simulink model "HouseHolderTransformTest"  (R2023b)
settings: Solver=VariableStepAuto  StartTime=0.0  StopTime=1  FixedStep=0.0038461538461538464  RelTol=1e-3
values from neighbouring files (symbols this model uses):
  A = [0.588528123101 -3.46944695195e-18 -8.67361737988e-19 0 0 6.93889390391e-18 6.93889390391e-18 6.93889390391e-18 1.38777878078e-17 0 0 6.93889390391e-18 ... (1040 elements, 260x4)]    [InitData.mat]
undefined symbols (not defined in the file or in its folder): FrameLength, NumOfAntennas
libraries: hdlsllib x5, dspstat3 x5
(part 2 of 2)

== system HouseHolderTransformTest/Subsystem/Subsystem3/vecnorm(A(k:end, k:end), 2, 1)/For Iterator Subsystem ==
  input : Inport
  N : Inport  Port=2
  2nd Norm : Subsystem
  Assignment : Assignment  IndexOptions=Index vector (port)  Indices=1  OutputSizes=1
  Constant : Constant  Value=zeros(1 , NumOfAntennas)
  For Iterator : ForIterator  IterationSource=external
  Selector : Selector  NumberOfDimensions=2  InputPortWidth=3  IndexOptions=Select all,Index vector (port)  Indices=[1 3],1  OutputSizes=1,1
  output : Outport
  wires:
  Assignment/1 -> output/1
  2nd Norm/1(output) -> Assignment/2
  Constant/1 -> Assignment/1
  N/1 -> For Iterator/1
  Selector/1 -> 2nd Norm/1(input)
  For Iterator/1 -> Selector/2, Assignment/3
  input/1 -> Selector/1

== system HouseHolderTransformTest/Subsystem/Subsystem4/BLOCK B/2nd Norm ==
  input : Inport
  Add : Sum
  Complex to Real-Imag : ComplexToRealImag
  Sqrt : Sqrt
  Square : Math  Operator=square  SignedPower=on  RndMeth=Zero
  Square1 : Math  Operator=square  SignedPower=on  RndMeth=Zero
  Sum of Elements : Sum  Inputs=+
  output : Outport
  wires:
  input/1 -> Complex to Real-Imag/1
  Complex to Real-Imag/2 -> Square1/1
  Sqrt/1 -> output/1
  Complex to Real-Imag/1 -> Square/1
  Square/1 -> Add/1
  Add/1 -> Sum of Elements/1
  Sum of Elements/1 -> Sqrt/1
  Square1/1 -> Add/2

== system HouseHolderTransformTest/Subsystem/Subsystem4/BLOCK B/If Action Subsystem ==
  norm : Inport
  x : Inport  Port=2
  Assignment : Assignment  IndexOptions=Index vector (dialog)  Indices=1  OutputSizes=1
  Divide : Subsystem  Tag=DecoupledSystem
  Divide1 : Subsystem  Tag=DecoupledSystem
  Selector : Selector  NumberOfDimensions=2  InputPortWidth=FrameLength  IndexOptions=Starting index (dialog),Index vector (dialog)  Indices=1,1  OutputSizes=1,1
  Sqrt : Sqrt
  Subsystem Reference : Subsystem  ReferencedSubsystem=CompAbs
  getU(1) : Subsystem
  u : Outport
  wires:
  getU(1)/1(u(1)) -> Subsystem Reference/1, Assignment/2  "u1"
  Assignment/1 -> Divide1/1(In1)
  Subsystem Reference/1 -> Sqrt/1
  Divide1/1(Out1) -> u/1
  Divide/1(Out1) -> Assignment/1, Selector/1
  norm/1 -> Divide/2(In2)
  x/1 -> Divide/1(In1)
  Selector/1 -> getU(1)/1(input)  "u1"
  Sqrt/1 -> Divide1/2(In2)

== system HouseHolderTransformTest/Subsystem/Subsystem4/BLOCK B/If Action Subsystem1 ==
  x : Inport
  Assignment : Assignment  IndexOptions=Index vector (dialog)  Indices=1  OutputSizes=1
  Constant : Constant  Value=sqrt(2)
  u : Outport
  wires:
  Assignment/1 -> u/1
  Constant/1 -> Assignment/2
  x/1 -> Assignment/1

== system HouseHolderTransformTest/Subsystem/Subsystem4/vecnorm(A(k:end, k:end), 2, 1)/For Iterator Subsystem ==
  input : Inport
  N : Inport  Port=2
  2nd Norm : Subsystem
  Assignment : Assignment  IndexOptions=Index vector (port)  Indices=1  OutputSizes=1
  Constant : Constant  Value=zeros(1 , NumOfAntennas)
  For Iterator : ForIterator  IterationSource=external
  Selector : Selector  NumberOfDimensions=2  InputPortWidth=3  IndexOptions=Select all,Index vector (port)  Indices=[1 3],1  OutputSizes=1,1
  output : Outport
  wires:
  input/1 -> Selector/1
  For Iterator/1 -> Assignment/3, Selector/2
  Selector/1 -> 2nd Norm/1(input)
  N/1 -> For Iterator/1
  Constant/1 -> Assignment/1
  2nd Norm/1(output) -> Assignment/2
  Assignment/1 -> output/1

== system HouseHolderTransformTest/For Iterator Subsystem1/Subsystem3/BLOCK B/If Action Subsystem/Divide ==
  In1 : Inport  LockScale=on
  In2 : Inport  Port=2  LockScale=on
  DTC_input_1 : DataTypeConversion  OutDataTypeStr=fixdt('double')  RndMeth=Nearest  SaturateOnIntegerOverflow=off  LockScale=on
  DTC_input_2 : DataTypeConversion  OutDataTypeStr=fixdt('double')  RndMeth=Nearest  SaturateOnIntegerOverflow=off  LockScale=on
  DTC_output_1 : DataTypeConversion  OutDataTypeStr=fixdt('double')  SaturateOnIntegerOverflow=off  RndMeth=Floor
  ReplicaOfSource : Product  Inputs=*/  RndMeth=Zero  SaturateOnIntegerOverflow=on
  Out1 : Outport  LockScale=on
  wires:
  ReplicaOfSource/1 -> DTC_output_1/1
  In1/1 -> DTC_input_1/1
  DTC_output_1/1 -> Out1/1
  In2/1 -> DTC_input_2/1
  DTC_input_2/1 -> ReplicaOfSource/2
  DTC_input_1/1 -> ReplicaOfSource/1

== system HouseHolderTransformTest/For Iterator Subsystem1/Subsystem3/BLOCK B/If Action Subsystem/Divide1 ==
  In1 : Inport  LockScale=on
  In2 : Inport  Port=2  LockScale=on
  DTC_input_1 : DataTypeConversion  OutDataTypeStr=fixdt('double')  RndMeth=Nearest  SaturateOnIntegerOverflow=off  LockScale=on
  DTC_input_2 : DataTypeConversion  OutDataTypeStr=fixdt('double')  RndMeth=Nearest  SaturateOnIntegerOverflow=off  LockScale=on
  DTC_output_1 : DataTypeConversion  OutDataTypeStr=fixdt('double')  SaturateOnIntegerOverflow=off  RndMeth=Floor
  ReplicaOfSource : Product  Inputs=*/  RndMeth=Zero  SaturateOnIntegerOverflow=on
  Out1 : Outport  LockScale=on
  wires:
  DTC_output_1/1 -> Out1/1
  In2/1 -> DTC_input_2/1
  In1/1 -> DTC_input_1/1
  DTC_input_1/1 -> ReplicaOfSource/1
  ReplicaOfSource/1 -> DTC_output_1/1
  DTC_input_2/1 -> ReplicaOfSource/2

== system HouseHolderTransformTest/For Iterator Subsystem1/Subsystem3/BLOCK B/If Action Subsystem/getU(1) ==
  input : Inport
  Add1 : Sum
  signNonComplex : Subsystem
  u(1) : Outport
  wires:
  signNonComplex/1(Out1) -> Add1/1
  input/1 -> Add1/2, signNonComplex/1(input)
  Add1/1 -> u(1)/1  "u(1)"

== system HouseHolderTransformTest/For Iterator Subsystem1/Subsystem3/vecnorm(A(k:end, k:end), 2, 1)/For Iterator Subsystem/2nd Norm ==
  input : Inport
  Add : Sum
  Complex to Real-Imag : ComplexToRealImag
  Sqrt : Sqrt
  Square : Math  Operator=square  SignedPower=on  RndMeth=Zero
  Square1 : Math  Operator=square  SignedPower=on  RndMeth=Zero
  Sum of Elements : Sum  Inputs=+
  output : Outport
  wires:
  input/1 -> Complex to Real-Imag/1
  Complex to Real-Imag/2 -> Square1/1
  Sqrt/1 -> output/1
  Complex to Real-Imag/1 -> Square/1
  Square/1 -> Add/1
  Add/1 -> Sum of Elements/1
  Sum of Elements/1 -> Sqrt/1
  Square1/1 -> Add/2

== system HouseHolderTransformTest/Subsystem/Subsystem1/BLOCK B/If Action Subsystem/Divide ==
  In1 : Inport  LockScale=on
  In2 : Inport  Port=2  LockScale=on
  DTC_input_1 : DataTypeConversion  OutDataTypeStr=fixdt('double')  RndMeth=Nearest  SaturateOnIntegerOverflow=off  LockScale=on
  DTC_input_2 : DataTypeConversion  OutDataTypeStr=fixdt('double')  RndMeth=Nearest  SaturateOnIntegerOverflow=off  LockScale=on
  DTC_output_1 : DataTypeConversion  OutDataTypeStr=fixdt('double')  SaturateOnIntegerOverflow=off  RndMeth=Floor
  ReplicaOfSource : Product  Inputs=*/  RndMeth=Zero  SaturateOnIntegerOverflow=on
  Out1 : Outport  LockScale=on
  wires:
  DTC_input_1/1 -> ReplicaOfSource/1
  DTC_input_2/1 -> ReplicaOfSource/2
  In2/1 -> DTC_input_2/1
  DTC_output_1/1 -> Out1/1
  In1/1 -> DTC_input_1/1
  ReplicaOfSource/1 -> DTC_output_1/1

== system HouseHolderTransformTest/Subsystem/Subsystem1/BLOCK B/If Action Subsystem/Divide1 ==
  In1 : Inport  LockScale=on
  In2 : Inport  Port=2  LockScale=on
  DTC_input_1 : DataTypeConversion  OutDataTypeStr=fixdt('double')  RndMeth=Nearest  SaturateOnIntegerOverflow=off  LockScale=on
  DTC_input_2 : DataTypeConversion  OutDataTypeStr=fixdt('double')  RndMeth=Nearest  SaturateOnIntegerOverflow=off  LockScale=on
  DTC_output_1 : DataTypeConversion  OutDataTypeStr=fixdt('double')  SaturateOnIntegerOverflow=off  RndMeth=Floor
  ReplicaOfSource : Product  Inputs=*/  RndMeth=Zero  SaturateOnIntegerOverflow=on
  Out1 : Outport  LockScale=on
  wires:
  DTC_input_2/1 -> ReplicaOfSource/2
  ReplicaOfSource/1 -> DTC_output_1/1
  DTC_input_1/1 -> ReplicaOfSource/1
  In1/1 -> DTC_input_1/1
  In2/1 -> DTC_input_2/1
  DTC_output_1/1 -> Out1/1

== system HouseHolderTransformTest/Subsystem/Subsystem1/BLOCK B/If Action Subsystem/getU(1) ==
  input : Inport
  Add1 : Sum
  signNonComplex : Subsystem
  u(1) : Outport
  wires:
  Add1/1 -> u(1)/1  "u(1)"
  input/1 -> signNonComplex/1(input), Add1/2
  signNonComplex/1(Out1) -> Add1/1

== system HouseHolderTransformTest/Subsystem/Subsystem1/vecnorm(A(k:end, k:end), 2, 1)/For Iterator Subsystem/2nd Norm ==
  input : Inport
  Add : Sum
  Complex to Real-Imag : ComplexToRealImag
  Sqrt : Sqrt
  Square : Math  Operator=square  SignedPower=on  RndMeth=Zero
  Square1 : Math  Operator=square  SignedPower=on  RndMeth=Zero
  Sum of Elements : Sum  Inputs=+
  output : Outport
  wires:
  Square1/1 -> Add/2
  Sum of Elements/1 -> Sqrt/1
  Add/1 -> Sum of Elements/1
  Square/1 -> Add/1
  Complex to Real-Imag/1 -> Square/1
  Sqrt/1 -> output/1
  Complex to Real-Imag/2 -> Square1/1
  input/1 -> Complex to Real-Imag/1

== system HouseHolderTransformTest/Subsystem/Subsystem2/BLOCK B/If Action Subsystem/Divide ==
  In1 : Inport  LockScale=on
  In2 : Inport  Port=2  LockScale=on
  DTC_input_1 : DataTypeConversion  OutDataTypeStr=fixdt('double')  RndMeth=Nearest  SaturateOnIntegerOverflow=off  LockScale=on
  DTC_input_2 : DataTypeConversion  OutDataTypeStr=fixdt('double')  RndMeth=Nearest  SaturateOnIntegerOverflow=off  LockScale=on
  DTC_output_1 : DataTypeConversion  OutDataTypeStr=fixdt('double')  SaturateOnIntegerOverflow=off  RndMeth=Floor
  ReplicaOfSource : Product  Inputs=*/  RndMeth=Zero  SaturateOnIntegerOverflow=on
  Out1 : Outport  LockScale=on
  wires:
  ReplicaOfSource/1 -> DTC_output_1/1
  In1/1 -> DTC_input_1/1
  DTC_output_1/1 -> Out1/1
  In2/1 -> DTC_input_2/1
  DTC_input_2/1 -> ReplicaOfSource/2
  DTC_input_1/1 -> ReplicaOfSource/1

== system HouseHolderTransformTest/Subsystem/Subsystem2/BLOCK B/If Action Subsystem/Divide1 ==
  In1 : Inport  LockScale=on
  In2 : Inport  Port=2  LockScale=on
  DTC_input_1 : DataTypeConversion  OutDataTypeStr=fixdt('double')  RndMeth=Nearest  SaturateOnIntegerOverflow=off  LockScale=on
  DTC_input_2 : DataTypeConversion  OutDataTypeStr=fixdt('double')  RndMeth=Nearest  SaturateOnIntegerOverflow=off  LockScale=on
  DTC_output_1 : DataTypeConversion  OutDataTypeStr=fixdt('double')  SaturateOnIntegerOverflow=off  RndMeth=Floor
  ReplicaOfSource : Product  Inputs=*/  RndMeth=Zero  SaturateOnIntegerOverflow=on
  Out1 : Outport  LockScale=on
  wires:
  DTC_output_1/1 -> Out1/1
  In2/1 -> DTC_input_2/1
  In1/1 -> DTC_input_1/1
  DTC_input_1/1 -> ReplicaOfSource/1
  ReplicaOfSource/1 -> DTC_output_1/1
  DTC_input_2/1 -> ReplicaOfSource/2

== system HouseHolderTransformTest/Subsystem/Subsystem2/BLOCK B/If Action Subsystem/getU(1) ==
  input : Inport
  Add1 : Sum
  signNonComplex : Subsystem
  u(1) : Outport
  wires:
  signNonComplex/1(Out1) -> Add1/1
  input/1 -> Add1/2, signNonComplex/1(input)
  Add1/1 -> u(1)/1  "u(1)"

== system HouseHolderTransformTest/Subsystem/Subsystem2/vecnorm(A(k:end, k:end), 2, 1)/For Iterator Subsystem/2nd Norm ==
  input : Inport
  Add : Sum
  Complex to Real-Imag : ComplexToRealImag
  Sqrt : Sqrt
  Square : Math  Operator=square  SignedPower=on  RndMeth=Zero
  Square1 : Math  Operator=square  SignedPower=on  RndMeth=Zero
  Sum of Elements : Sum  Inputs=+
  output : Outport
  wires:
  input/1 -> Complex to Real-Imag/1
  Complex to Real-Imag/2 -> Square1/1
  Sqrt/1 -> output/1
  Complex to Real-Imag/1 -> Square/1
  Square/1 -> Add/1
  Add/1 -> Sum of Elements/1
  Sum of Elements/1 -> Sqrt/1
  Square1/1 -> Add/2

== system HouseHolderTransformTest/Subsystem/Subsystem3/BLOCK B/If Action Subsystem/Divide ==
  In1 : Inport  LockScale=on
  In2 : Inport  Port=2  LockScale=on
  DTC_input_1 : DataTypeConversion  OutDataTypeStr=fixdt('double')  RndMeth=Nearest  SaturateOnIntegerOverflow=off  LockScale=on
  DTC_input_2 : DataTypeConversion  OutDataTypeStr=fixdt('double')  RndMeth=Nearest  SaturateOnIntegerOverflow=off  LockScale=on
  DTC_output_1 : DataTypeConversion  OutDataTypeStr=fixdt('double')  SaturateOnIntegerOverflow=off  RndMeth=Floor
  ReplicaOfSource : Product  Inputs=*/  RndMeth=Zero  SaturateOnIntegerOverflow=on
  Out1 : Outport  LockScale=on
  wires:
  ReplicaOfSource/1 -> DTC_output_1/1
  In1/1 -> DTC_input_1/1
  DTC_output_1/1 -> Out1/1
  In2/1 -> DTC_input_2/1
  DTC_input_2/1 -> ReplicaOfSource/2
  DTC_input_1/1 -> ReplicaOfSource/1

== system HouseHolderTransformTest/Subsystem/Subsystem3/BLOCK B/If Action Subsystem/Divide1 ==
  In1 : Inport  LockScale=on
  In2 : Inport  Port=2  LockScale=on
  DTC_input_1 : DataTypeConversion  OutDataTypeStr=fixdt('double')  RndMeth=Nearest  SaturateOnIntegerOverflow=off  LockScale=on
  DTC_input_2 : DataTypeConversion  OutDataTypeStr=fixdt('double')  RndMeth=Nearest  SaturateOnIntegerOverflow=off  LockScale=on
  DTC_output_1 : DataTypeConversion  OutDataTypeStr=fixdt('double')  SaturateOnIntegerOverflow=off  RndMeth=Floor
  ReplicaOfSource : Product  Inputs=*/  RndMeth=Zero  SaturateOnIntegerOverflow=on
  Out1 : Outport  LockScale=on
  wires:
  DTC_output_1/1 -> Out1/1
  In2/1 -> DTC_input_2/1
  In1/1 -> DTC_input_1/1
  DTC_input_1/1 -> ReplicaOfSource/1
  ReplicaOfSource/1 -> DTC_output_1/1
  DTC_input_2/1 -> ReplicaOfSource/2

== system HouseHolderTransformTest/Subsystem/Subsystem3/BLOCK B/If Action Subsystem/getU(1) ==
  input : Inport
  Add1 : Sum
  signNonComplex : Subsystem
  u(1) : Outport
  wires:
  signNonComplex/1(Out1) -> Add1/1
  input/1 -> Add1/2, signNonComplex/1(input)
  Add1/1 -> u(1)/1  "u(1)"

== system HouseHolderTransformTest/Subsystem/Subsystem3/vecnorm(A(k:end, k:end), 2, 1)/For Iterator Subsystem/2nd Norm ==
  input : Inport
  Add : Sum
  Complex to Real-Imag : ComplexToRealImag
  Sqrt : Sqrt
  Square : Math  Operator=square  SignedPower=on  RndMeth=Zero
  Square1 : Math  Operator=square  SignedPower=on  RndMeth=Zero
  Sum of Elements : Sum  Inputs=+
  output : Outport
  wires:
  input/1 -> Complex to Real-Imag/1
  Complex to Real-Imag/2 -> Square1/1
  Sqrt/1 -> output/1
  Complex to Real-Imag/1 -> Square/1
  Square/1 -> Add/1
  Add/1 -> Sum of Elements/1
  Sum of Elements/1 -> Sqrt/1
  Square1/1 -> Add/2

== system HouseHolderTransformTest/Subsystem/Subsystem4/BLOCK B/If Action Subsystem/Divide ==
  In1 : Inport  LockScale=on
  In2 : Inport  Port=2  LockScale=on
  DTC_input_1 : DataTypeConversion  OutDataTypeStr=fixdt('double')  RndMeth=Nearest  SaturateOnIntegerOverflow=off  LockScale=on
  DTC_input_2 : DataTypeConversion  OutDataTypeStr=fixdt('double')  RndMeth=Nearest  SaturateOnIntegerOverflow=off  LockScale=on
  DTC_output_1 : DataTypeConversion  OutDataTypeStr=fixdt('double')  SaturateOnIntegerOverflow=off  RndMeth=Floor
  ReplicaOfSource : Product  Inputs=*/  RndMeth=Zero  SaturateOnIntegerOverflow=on
  Out1 : Outport  LockScale=on
  wires:
  DTC_input_1/1 -> ReplicaOfSource/1
  DTC_input_2/1 -> ReplicaOfSource/2
  In2/1 -> DTC_input_2/1
  DTC_output_1/1 -> Out1/1
  In1/1 -> DTC_input_1/1
  ReplicaOfSource/1 -> DTC_output_1/1

== system HouseHolderTransformTest/Subsystem/Subsystem4/BLOCK B/If Action Subsystem/Divide1 ==
  In1 : Inport  LockScale=on
  In2 : Inport  Port=2  LockScale=on
  DTC_input_1 : DataTypeConversion  OutDataTypeStr=fixdt('double')  RndMeth=Nearest  SaturateOnIntegerOverflow=off  LockScale=on
  DTC_input_2 : DataTypeConversion  OutDataTypeStr=fixdt('double')  RndMeth=Nearest  SaturateOnIntegerOverflow=off  LockScale=on
  DTC_output_1 : DataTypeConversion  OutDataTypeStr=fixdt('double')  SaturateOnIntegerOverflow=off  RndMeth=Floor
  ReplicaOfSource : Product  Inputs=*/  RndMeth=Zero  SaturateOnIntegerOverflow=on
  Out1 : Outport  LockScale=on
  wires:
  DTC_input_2/1 -> ReplicaOfSource/2
  ReplicaOfSource/1 -> DTC_output_1/1
  DTC_input_1/1 -> ReplicaOfSource/1
  In1/1 -> DTC_input_1/1
  In2/1 -> DTC_input_2/1
  DTC_output_1/1 -> Out1/1

== system HouseHolderTransformTest/Subsystem/Subsystem4/BLOCK B/If Action Subsystem/getU(1) ==
  input : Inport
  Add1 : Sum
  signNonComplex : Subsystem
  u(1) : Outport
  wires:
  Add1/1 -> u(1)/1  "u(1)"
  input/1 -> signNonComplex/1(input), Add1/2
  signNonComplex/1(Out1) -> Add1/1

== system HouseHolderTransformTest/Subsystem/Subsystem4/vecnorm(A(k:end, k:end), 2, 1)/For Iterator Subsystem/2nd Norm ==
  input : Inport
  Add : Sum
  Complex to Real-Imag : ComplexToRealImag
  Sqrt : Sqrt
  Square : Math  Operator=square  SignedPower=on  RndMeth=Zero
  Square1 : Math  Operator=square  SignedPower=on  RndMeth=Zero
  Sum of Elements : Sum  Inputs=+
  output : Outport
  wires:
  Square1/1 -> Add/2
  Sum of Elements/1 -> Sqrt/1
  Add/1 -> Sum of Elements/1
  Square/1 -> Add/1
  Complex to Real-Imag/1 -> Square/1
  Sqrt/1 -> output/1
  Complex to Real-Imag/2 -> Square1/1
  input/1 -> Complex to Real-Imag/1

== system HouseHolderTransformTest/For Iterator Subsystem1/Subsystem3/BLOCK B/If Action Subsystem/getU(1)/signNonComplex ==
  input : Inport
  Add : Sum
  Compare To Constant : hdlsllib/Logic and Bit Operations/Compare To Constant  relop===  const=0  OutDataTypeStr=boolean
  Divide : Subsystem  Tag=DecoupledSystem
  Subsystem Reference : Subsystem  ReferencedSubsystem=CompAbs
  Out1 : Outport
  wires:
  Subsystem Reference/1 -> Divide/2(In2)
  input/1 -> Subsystem Reference/1, Divide/1(In1)
  Add/1 -> Out1/1
  Compare To Constant/1 -> Add/1
  Divide/1(Out1) -> Add/2, Compare To Constant/1

== system HouseHolderTransformTest/Subsystem/Subsystem1/BLOCK B/If Action Subsystem/getU(1)/signNonComplex ==
  input : Inport
  Add : Sum
  Compare To Constant : hdlsllib/Logic and Bit Operations/Compare To Constant  relop===  const=0  OutDataTypeStr=boolean
  Divide : Subsystem  Tag=DecoupledSystem
  Subsystem Reference : Subsystem  ReferencedSubsystem=CompAbs
  Out1 : Outport
  wires:
  Divide/1(Out1) -> Compare To Constant/1, Add/2
  Compare To Constant/1 -> Add/1
  Add/1 -> Out1/1
  input/1 -> Divide/1(In1), Subsystem Reference/1
  Subsystem Reference/1 -> Divide/2(In2)

== system HouseHolderTransformTest/Subsystem/Subsystem2/BLOCK B/If Action Subsystem/getU(1)/signNonComplex ==
  input : Inport
  Add : Sum
  Compare To Constant : hdlsllib/Logic and Bit Operations/Compare To Constant  relop===  const=0  OutDataTypeStr=boolean
  Divide : Subsystem  Tag=DecoupledSystem
  Subsystem Reference : Subsystem  ReferencedSubsystem=CompAbs
  Out1 : Outport
  wires:
  Subsystem Reference/1 -> Divide/2(In2)
  input/1 -> Subsystem Reference/1, Divide/1(In1)
  Add/1 -> Out1/1
  Compare To Constant/1 -> Add/1
  Divide/1(Out1) -> Add/2, Compare To Constant/1

== system HouseHolderTransformTest/Subsystem/Subsystem3/BLOCK B/If Action Subsystem/getU(1)/signNonComplex ==
  input : Inport
  Add : Sum
  Compare To Constant : hdlsllib/Logic and Bit Operations/Compare To Constant  relop===  const=0  OutDataTypeStr=boolean
  Divide : Subsystem  Tag=DecoupledSystem
  Subsystem Reference : Subsystem  ReferencedSubsystem=CompAbs
  Out1 : Outport
  wires:
  Subsystem Reference/1 -> Divide/2(In2)
  input/1 -> Subsystem Reference/1, Divide/1(In1)
  Add/1 -> Out1/1
  Compare To Constant/1 -> Add/1
  Divide/1(Out1) -> Add/2, Compare To Constant/1

== system HouseHolderTransformTest/Subsystem/Subsystem4/BLOCK B/If Action Subsystem/getU(1)/signNonComplex ==
  input : Inport
  Add : Sum
  Compare To Constant : hdlsllib/Logic and Bit Operations/Compare To Constant  relop===  const=0  OutDataTypeStr=boolean
  Divide : Subsystem  Tag=DecoupledSystem
  Subsystem Reference : Subsystem  ReferencedSubsystem=CompAbs
  Out1 : Outport
  wires:
  Divide/1(Out1) -> Compare To Constant/1, Add/2
  Compare To Constant/1 -> Add/1
  Add/1 -> Out1/1
  input/1 -> Divide/1(In1), Subsystem Reference/1
  Subsystem Reference/1 -> Divide/2(In2)

== system HouseHolderTransformTest/For Iterator Subsystem1/Subsystem3/BLOCK B/If Action Subsystem/getU(1)/signNonComplex/Divide ==
  In1 : Inport  LockScale=on
  In2 : Inport  Port=2  LockScale=on
  DTC_input_1 : DataTypeConversion  OutDataTypeStr=fixdt('double')  RndMeth=Nearest  SaturateOnIntegerOverflow=off  LockScale=on
  DTC_input_2 : DataTypeConversion  OutDataTypeStr=fixdt('double')  RndMeth=Nearest  SaturateOnIntegerOverflow=off  LockScale=on
  DTC_output_1 : DataTypeConversion  OutDataTypeStr=fixdt('double')  SaturateOnIntegerOverflow=off  RndMeth=Floor
  ReplicaOfSource : Product  Inputs=*/  RndMeth=Zero  SaturateOnIntegerOverflow=on
  Out1 : Outport  LockScale=on
  wires:
  In1/1 -> DTC_input_1/1
  In2/1 -> DTC_input_2/1
  DTC_input_2/1 -> ReplicaOfSource/2
  DTC_output_1/1 -> Out1/1
  ReplicaOfSource/1 -> DTC_output_1/1
  DTC_input_1/1 -> ReplicaOfSource/1

== system HouseHolderTransformTest/Subsystem/Subsystem1/BLOCK B/If Action Subsystem/getU(1)/signNonComplex/Divide ==
  In1 : Inport  LockScale=on
  In2 : Inport  Port=2  LockScale=on
  DTC_input_1 : DataTypeConversion  OutDataTypeStr=fixdt('double')  RndMeth=Nearest  SaturateOnIntegerOverflow=off  LockScale=on
  DTC_input_2 : DataTypeConversion  OutDataTypeStr=fixdt('double')  RndMeth=Nearest  SaturateOnIntegerOverflow=off  LockScale=on
  DTC_output_1 : DataTypeConversion  OutDataTypeStr=fixdt('double')  SaturateOnIntegerOverflow=off  RndMeth=Floor
  ReplicaOfSource : Product  Inputs=*/  RndMeth=Zero  SaturateOnIntegerOverflow=on
  Out1 : Outport  LockScale=on
  wires:
  DTC_input_1/1 -> ReplicaOfSource/1
  ReplicaOfSource/1 -> DTC_output_1/1
  DTC_output_1/1 -> Out1/1
  DTC_input_2/1 -> ReplicaOfSource/2
  In2/1 -> DTC_input_2/1
  In1/1 -> DTC_input_1/1

== system HouseHolderTransformTest/Subsystem/Subsystem2/BLOCK B/If Action Subsystem/getU(1)/signNonComplex/Divide ==
  In1 : Inport  LockScale=on
  In2 : Inport  Port=2  LockScale=on
  DTC_input_1 : DataTypeConversion  OutDataTypeStr=fixdt('double')  RndMeth=Nearest  SaturateOnIntegerOverflow=off  LockScale=on
  DTC_input_2 : DataTypeConversion  OutDataTypeStr=fixdt('double')  RndMeth=Nearest  SaturateOnIntegerOverflow=off  LockScale=on
  DTC_output_1 : DataTypeConversion  OutDataTypeStr=fixdt('double')  SaturateOnIntegerOverflow=off  RndMeth=Floor
  ReplicaOfSource : Product  Inputs=*/  RndMeth=Zero  SaturateOnIntegerOverflow=on
  Out1 : Outport  LockScale=on
  wires:
  In1/1 -> DTC_input_1/1
  In2/1 -> DTC_input_2/1
  DTC_input_2/1 -> ReplicaOfSource/2
  DTC_output_1/1 -> Out1/1
  ReplicaOfSource/1 -> DTC_output_1/1
  DTC_input_1/1 -> ReplicaOfSource/1

== system HouseHolderTransformTest/Subsystem/Subsystem3/BLOCK B/If Action Subsystem/getU(1)/signNonComplex/Divide ==
  In1 : Inport  LockScale=on
  In2 : Inport  Port=2  LockScale=on
  DTC_input_1 : DataTypeConversion  OutDataTypeStr=fixdt('double')  RndMeth=Nearest  SaturateOnIntegerOverflow=off  LockScale=on
  DTC_input_2 : DataTypeConversion  OutDataTypeStr=fixdt('double')  RndMeth=Nearest  SaturateOnIntegerOverflow=off  LockScale=on
  DTC_output_1 : DataTypeConversion  OutDataTypeStr=fixdt('double')  SaturateOnIntegerOverflow=off  RndMeth=Floor
  ReplicaOfSource : Product  Inputs=*/  RndMeth=Zero  SaturateOnIntegerOverflow=on
  Out1 : Outport  LockScale=on
  wires:
  In1/1 -> DTC_input_1/1
  In2/1 -> DTC_input_2/1
  DTC_input_2/1 -> ReplicaOfSource/2
  DTC_output_1/1 -> Out1/1
  ReplicaOfSource/1 -> DTC_output_1/1
  DTC_input_1/1 -> ReplicaOfSource/1

== system HouseHolderTransformTest/Subsystem/Subsystem4/BLOCK B/If Action Subsystem/getU(1)/signNonComplex/Divide ==
  In1 : Inport  LockScale=on
  In2 : Inport  Port=2  LockScale=on
  DTC_input_1 : DataTypeConversion  OutDataTypeStr=fixdt('double')  RndMeth=Nearest  SaturateOnIntegerOverflow=off  LockScale=on
  DTC_input_2 : DataTypeConversion  OutDataTypeStr=fixdt('double')  RndMeth=Nearest  SaturateOnIntegerOverflow=off  LockScale=on
  DTC_output_1 : DataTypeConversion  OutDataTypeStr=fixdt('double')  SaturateOnIntegerOverflow=off  RndMeth=Floor
  ReplicaOfSource : Product  Inputs=*/  RndMeth=Zero  SaturateOnIntegerOverflow=on
  Out1 : Outport  LockScale=on
  wires:
  DTC_input_1/1 -> ReplicaOfSource/1
  ReplicaOfSource/1 -> DTC_output_1/1
  DTC_output_1/1 -> Out1/1
  DTC_input_2/1 -> ReplicaOfSource/2
  In2/1 -> DTC_input_2/1
  In1/1 -> DTC_input_1/1

== matlab function HouseHolderTransformTest/MATLAB Function ==
  data: A output; A input; p output
function [A, p] = stepImpl(A)
    %#codegen

    [m, n] = size(A);
    p = int32(1:n);

    % Define Householder transformation function
    H = @(u, x) x - u * (u' * x);

    % Main loop
    for k = 1:min(m, n)
        % Find column with maximum norm for column pivoting
        [~, idx] = max(vecnorm(A(k:end, k:end), 2, 1));
        idx = int32(idx + k - 1); % Ensure integer type for HDL code generation
        if idx ~= k
            % Swap columns in A and p
            A(:, [k, idx]) = A(:, [idx, k]);
            % p([k, idx]) = p([idx, k]);
        end

        % Apply Householder transformation
        x = A(k:m, k);
        h = housegen(x);
        A(k:m, k:n) = H(h, A(k:m, k:n));
    end
      
end

== matlab function HouseHolderTransformTest/Subsystem/Subsystem3/BLOCK A/MATLAB Function ==
  data: A input; idx input; A output; k input
function A = swap(A , idx ,  k )
% %#codegen
 A(:, [k, idx]) = A(:, [idx, k]);
end

== matlab function HouseHolderTransformTest/Subsystem/Subsystem3/MATLAB Function ==
  data: u input; y output size=[260 4]; x input
function y = fcn(u, x)
    y = x - u*(u'*x);
end

== matlab function HouseHolderTransformTest/For Iterator Subsystem1/Subsystem3/BLOCK A/MATLAB Function ==
  data: A input; idx input; A output; k input
function A = swap(A , idx ,  k )
% %#codegen
 A(:, [k, idx]) = A(:, [idx, k]);
end

== matlab function HouseHolderTransformTest/For Iterator Subsystem1/Subsystem3/MATLAB Function ==
  data: u input; y output size=[260 4]; x input
function y = fcn(u, x)
    y = x - u*(u'*x);
end

== matlab function HouseHolderTransformTest/Subsystem/Subsystem1/BLOCK A/MATLAB Function ==
  data: A input; idx input; A output; k input
function A = swap(A , idx ,  k )
% %#codegen
 A(:, [k, idx]) = A(:, [idx, k]);
end

== matlab function HouseHolderTransformTest/Subsystem/Subsystem1/MATLAB Function ==
  data: u input; y output size=[260 4]; x input
function y = fcn(u, x)
    y = x - u*(u'*x);
end

== matlab function HouseHolderTransformTest/Subsystem/Subsystem2/BLOCK A/MATLAB Function ==
  data: A input; idx input; A output; k input
function A = swap(A , idx ,  k )
% %#codegen
 A(:, [k, idx]) = A(:, [idx, k]);
end

== matlab function HouseHolderTransformTest/Subsystem/Subsystem2/MATLAB Function ==
  data: u input; y output size=[260 4]; x input
function y = fcn(u, x)
    y = x - u*(u'*x);
end

== matlab function HouseHolderTransformTest/Subsystem/Subsystem4/BLOCK A/MATLAB Function ==
  data: A input; idx input; A output; k input
function A = swap(A , idx ,  k )
% %#codegen
 A(:, [k, idx]) = A(:, [idx, k]);
end

== matlab function HouseHolderTransformTest/Subsystem/Subsystem4/MATLAB Function ==
  data: u input; y output size=[260 4]; x input
function y = fcn(u, x)
    y = x - u*(u'*x);
end
